simulink model "embedded_with_reshape"  (Simulink 7.9)
settings: Solver=ode3  StartTime=0.0  StopTime=10.0  FixedStep=1  RelTol=1e-3
settings Model: Creator=Harmon S. Nine  LastModifiedBy=hnine
settings DataIOCC: SaveFormat=Structure
settings DebuggingCC: FcnCallInpInsideContextMsg=Use local settings  StrictBusMsg=Warning
settings SFSimCC: SimParseCustomCode=off
settings GRTTargetCC: CombineOutputUpdateFcns=off  GRTInterface=on

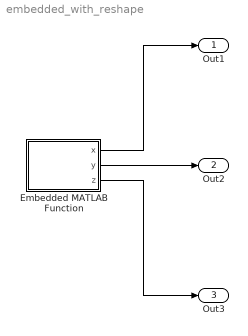
== system embedded_with_reshape ==
  Embedded MATLAB Function : MATLAB Function  TreatAsAtomicUnit=on
  Out1 : Outport
  Out2 : Outport  Port=2
  Out3 : Outport  Port=3
  wires:
  Embedded MATLAB Function/2(y) -> Out2/1
  Embedded MATLAB Function/1(x) -> Out1/1
  Embedded MATLAB Function/3(z) -> Out3/1

== matlab function Embedded MATLAB Function ==
  data: x output double; y output double; z output double
function [x,y,z] = fcn()
%#eml

testvalue = reshape( [ 1 2 3 4 5 6 7 8 9 10 11 12 13 14 15 16 17 18 19 20 21 22 23 24 25 26 27 28 29 30 31 32 33 34 35 36 ], [3 2 3 2] );

x = reshape( testvalue( :, 2, :, 1 ), [3 , 3] );
y = testvalue( 2, 2, 2, 2 );
z = testvalue( 2, :, 2, 1 );
